simulink model "dc_transient"  (R2018a)
settings: Solver=VariableStepAuto  StartTime=0.0  StopTime=2  RelTol=1e-3
libraries: powerlib x19
settings Model: Creator=Sadat Zubin Shah  LastModifiedBy=Sadat Zubin Shah

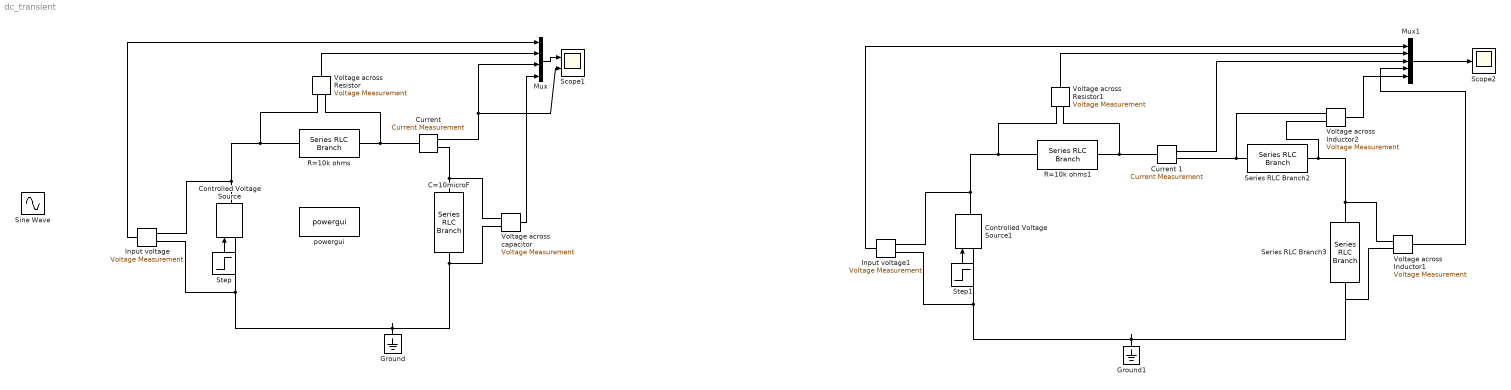
== system dc_transient ==
  C=10microF : powerlib/Elements/Series RLC Branch  LConnTagsString=__new0  RConnTagsString=__new0  BranchType=C  Resistance=1  Inductance=0.1  SetiL0=off  InitialCurrent=0  Capacitance=10e-6  Setx0=off  InitialVoltage=0  Measurements=None
  Controlled Voltage Source : powerlib/Electrical Sources/Controlled Voltage Source  Initialize=off  Source_Type=AC  Amplitude=0  Phase=0  Frequency=0  Measurements=None
  Controlled Voltage Source1 : powerlib/Electrical Sources/Controlled Voltage Source  Initialize=off  Source_Type=AC  Amplitude=0  Phase=0  Frequency=0  Measurements=None
  "Current " : powerlib/Measurements/Current Measurement  PhasorSimulation=off  OutputType=Complex  PSBequivalent=0
  Current 1 : powerlib/Measurements/Current Measurement  PhasorSimulation=off  OutputType=Complex  PSBequivalent=0
  Ground : powerlib/Elements/Ground  LConnTagsString=a
  Ground1 : powerlib/Elements/Ground  LConnTagsString=a
  Input voltage : powerlib/Measurements/Voltage Measurement  PhasorSimulation=off  OutputType=Complex  PSBequivalent=0
  Input voltage1 : powerlib/Measurements/Voltage Measurement  PhasorSimulation=off  OutputType=Complex  PSBequivalent=0
  Mux : Mux
  Mux1 : Mux  Inputs=5
  R=10k ohms : powerlib/Elements/Series RLC Branch  LConnTagsString=__new0  RConnTagsString=__new0  BranchType=R  Resistance=10000  Inductance=1e-3  SetiL0=off  InitialCurrent=0  Capacitance=1e-6  Setx0=off  InitialVoltage=0  Measurements=None
  R=10k ohms1 : powerlib/Elements/Series RLC Branch  LConnTagsString=__new0  RConnTagsString=__new0  BranchType=R  Resistance=10  Inductance=1e-3  SetiL0=off  InitialCurrent=0  Capacitance=1e-6  Setx0=off  InitialVoltage=0  Measurements=None
  Scope1 : Scope  NumInputPorts=2
  Scope2 : Scope
  Series RLC Branch2 : powerlib/Elements/Series RLC Branch  LConnTagsString=__new0  RConnTagsString=__new0  BranchType=L  Resistance=1  Inductance=1  SetiL0=off  InitialCurrent=0  Capacitance=10e-6  Setx0=off  InitialVoltage=0  Measurements=None
  Series RLC Branch3 : powerlib/Elements/Series RLC Branch  LConnTagsString=__new0  RConnTagsString=__new0  BranchType=C  Resistance=1  Inductance=0.1  SetiL0=off  InitialCurrent=0  Capacitance=10e-6  Setx0=off  InitialVoltage=0  Measurements=None
  Sine Wave : Sin  SampleTime=0
  Step : Step  Before=10  After=0  SampleTime=0.01
  Step1 : Step  Before=10  After=0  SampleTime=0.01
  Voltage across Inductor1 : powerlib/Measurements/Voltage Measurement  PhasorSimulation=off  OutputType=Complex  PSBequivalent=0
  Voltage across Inductor2 : powerlib/Measurements/Voltage Measurement  PhasorSimulation=off  OutputType=Complex  PSBequivalent=0
  Voltage across Resistor : powerlib/Measurements/Voltage Measurement  PhasorSimulation=off  OutputType=Complex  PSBequivalent=0
  Voltage across Resistor1 : powerlib/Measurements/Voltage Measurement  PhasorSimulation=off  OutputType=Complex  PSBequivalent=0
  Voltage across capacitor : powerlib/Measurements/Voltage Measurement  PhasorSimulation=off  OutputType=Complex  PSBequivalent=0
  powergui : powerlib/powergui  Priority=1  SimulationMode=Discrete  SampleTime=50e-6  frequency=60  Iterations=50  frequencyindice=0  Pbase=100e6  ErrMax=1e-4  UnitsV=kV  UnitsW=MW  buscounter=0  FunctionMessages=off  echomessages=off  EnableUseOfTLC=off  CurrentSourceSwitches=off  DisableSnubberDevices=off  DisableRonSwitches=off  DisableVfSwitches=off  DisplayEquations=off  SolverType=Tustin/Backward Euler (TBE)  Interpol=off  ExternalGateDelay=off  methode=off  Ts=100  x0status=blocks  SPID=on  SwTol=0  HookPort=off  RestoreLinks=warning  ResistiveCurrentMeasurement=off  Frange=[0:2:500]  Ylog=off  Xlog=on  ShowGrid=off  save=off  variable=ZData  structure=0  ZoomFFT=off  StartTime=0.0  cycles=1  DisplayStyle=1  fundamental=60  FreqAxis=off  MaxFrequency=1000  frequencyindicesteady=1  RmsSteady=1  display=off
  wires:
  Step/1 -> Controlled Voltage Source/1
  Input voltage/1 -> Mux/1
  Voltage across Resistor/1 -> Mux/2
  Voltage across capacitor/1 -> Mux/4
  "Current "/1 -> Scope1/2, Mux/3
  Mux/1 -> Scope1/1
  Mux1/1 -> Scope2/1
  Current 1/1 -> Mux1/3
  Voltage across Inductor1/1 -> Mux1/4
  Voltage across Resistor1/1 -> Mux1/2
  Input voltage1/1 -> Mux1/1
  Step1/1 -> Controlled Voltage Source1/1
  Voltage across Inductor2/1 -> Mux1/5
  connections:
  Ground/LConn1 -- Voltage across capacitor/LConn2 -- C=10microF/RConn1 -- Input voltage/LConn2 -- Controlled Voltage Source/LConn1
  R=10k ohms/LConn1 -- Voltage across Resistor/LConn1 -- Input voltage/LConn1 -- Controlled Voltage Source/RConn1
  "Current "/LConn1 -- Voltage across Resistor/LConn2 -- R=10k ohms/RConn1
  C=10microF/LConn1 -- Voltage across capacitor/LConn1 -- "Current "/RConn1
  Ground1/LConn1 -- Voltage across Inductor1/LConn2 -- Series RLC Branch3/RConn1 -- Controlled Voltage Source1/LConn1 -- Input voltage1/LConn2
  R=10k ohms1/LConn1 -- Controlled Voltage Source1/RConn1 -- Input voltage1/LConn1 -- Voltage across Resistor1/LConn1
  Current 1/LConn1 -- R=10k ohms1/RConn1 -- Voltage across Resistor1/LConn2
  Series RLC Branch2/LConn1 -- Voltage across Inductor2/LConn1 -- Current 1/RConn1
  Series RLC Branch3/LConn1 -- Voltage across Inductor1/LConn1 -- Voltage across Inductor2/LConn2 -- Series RLC Branch2/RConn1
